simulink model "InvertedPendulum"  (R2017a)
settings: Solver=VariableStepAuto  StartTime=0.0  StopTime=10.0  RelTol=1e-3
settings Model: Creator=aposad31  LastModifiedBy=Asus

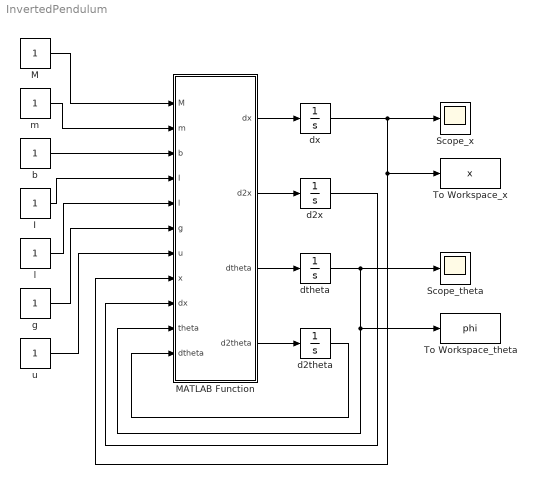
== system InvertedPendulum ==
  I : Constant
  M : Constant
  MATLAB Function : MATLAB Function  TreatAsAtomicUnit=on
  Scope_theta : Scope
  Scope_x : Scope
  To Workspace_theta : ToWorkspace  VariableName=phi  SaveFormat=Timeseries  SampleTime=-1
  To Workspace_x : ToWorkspace  VariableName=x  SaveFormat=Timeseries  SampleTime=-1
  b : Constant
  d2theta : Integrator
  d2x : Integrator
  dtheta : Integrator
  dx : Integrator
  g : Constant
  l : Constant
  m : Constant
  u : Constant
  wires:
  M/1 -> MATLAB Function/1(M)
  m/1 -> MATLAB Function/2(m)
  b/1 -> MATLAB Function/3(b)
  I/1 -> MATLAB Function/4(I)
  l/1 -> MATLAB Function/5(l)
  g/1 -> MATLAB Function/6(g)
  u/1 -> MATLAB Function/7(u)
  MATLAB Function/1(dx) -> dx/1
  MATLAB Function/2(d2x) -> d2x/1
  MATLAB Function/3(dtheta) -> dtheta/1
  MATLAB Function/4(d2theta) -> d2theta/1
  dx/1 -> Scope_x/1, To Workspace_x/1, MATLAB Function/8(x)
  d2x/1 -> MATLAB Function/9("dx ")
  dtheta/1 -> Scope_theta/1, To Workspace_theta/1, MATLAB Function/10(theta)
  d2theta/1 -> MATLAB Function/11("dtheta ")

== matlab function InvertedPendulum/MATLAB Function ==
  data: M input; m input; b input; I input; l input; g input; u input; dx output; x input; dx input; theta input; dtheta input; d2x output; dtheta output; d2theta output
function [dx, d2x, dtheta, d2theta] = fcn(M, m, b, I, l, g, u, x, dx, theta, dtheta)
    denominator = (M+m)*(I+m*l^2)-m^2*l^2*cos(theta)^2;
    dx = dx;
    d2x = ((I+m*l^2)*u-(I+m*l^2)*b*dx+m^2*l^2*g*sin(theta)*cos(theta)-(I+m*l^2)*dtheta^2*sin(theta))/denominator;
    dtheta = dtheta;
    d2theta = (-m*l*cos(theta)*u+m*l*b*cos(theta)*dx+m^2*l^2*dtheta^2*sin(theta)*cos(theta)-(M+m)*m*g*l*sin(theta))/denominator;
end
